simulink model "thermalBuilding3221"  (Simulink 8.3)
settings: Solver=ode5  StartTime=0.0  StopTime=24  FixedStep=stepSize  RelTol=1e-3
model workspace: external: MAT-File D:\PROGRAMMING-IDEs\MATLAB\1WORKSPACE\1_Projects\Smart-Building\WIN/Data/wsVars/thermalBuilding3221WS.mat (data not in the file)
undefined symbols (not defined in the file): Ca, Ceq, cost, DiscIntNeverNeededParam, Mafc, Mafh, Req, Rwall, stepSize, TAout, TCooler, THeater, TInit, TSet1, TSet2, TSet3
libraries: dspsigops x1
(part 1 of 2)
settings Model: Creator=salanda  LastModifiedBy=salanda
settings DataIOCC: SignalLoggingSaveFormat=Dataset
settings DebuggingCC: UnderspecifiedInitializationDetection=Simplified  ParameterPrecisionLossMsg=none  StateNameClashWarn=none
settings GRTTargetCC: CombineOutputUpdateFcns=on  GRTInterface=off

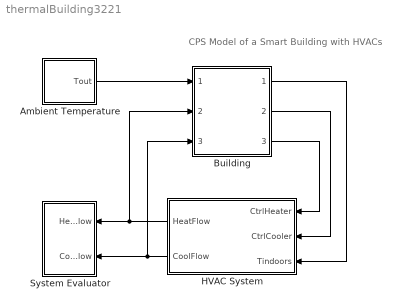
== system thermalBuilding3221 ==
  note: CPS Model of a Smart Building with HVACs
  Ambient Temperature : Subsystem
  Building : Subsystem
      mask Display: image(imread('building.png'))
  HVAC System : Subsystem
  System Evaluator : Subsystem
  wires:
  Ambient Temperature/1(Tout) -> Building/1(Outdoor Temp)
  HVAC System/1(HeatFlow) -> System Evaluator/1(HeatFlow), Building/2(HeatFlow)
  HVAC System/2(CoolFlow) -> System Evaluator/2(CoolFlow), Building/3(CoolFlow)
  Building/3(Heater  On/Off) -> HVAC System/1(CtrlHeater)
  Building/2(Cooler  On/Off) -> HVAC System/2(CtrlCooler)
  Building/1(Tindoors) -> HVAC System/3(Tindoors)

== system thermalBuilding3221/Ambient Temperature ==
  Avg Outdoor Temp : Constant  Value=TAout
  Daily Temp Variation : Sin  Amplitude=15  Frequency=2*pi/24  SampleTime=0
  Sum1 : Sum  Inputs=|++  SaturateOnIntegerOverflow=on  InputSameDT=on  OutDataTypeStr=Inherit: Same as first input
  Tout : Outport
  wires:
  Daily Temp Variation/1 -> Sum1/2
  Avg Outdoor Temp/1 -> Sum1/1
  Sum1/1 -> Tout/1

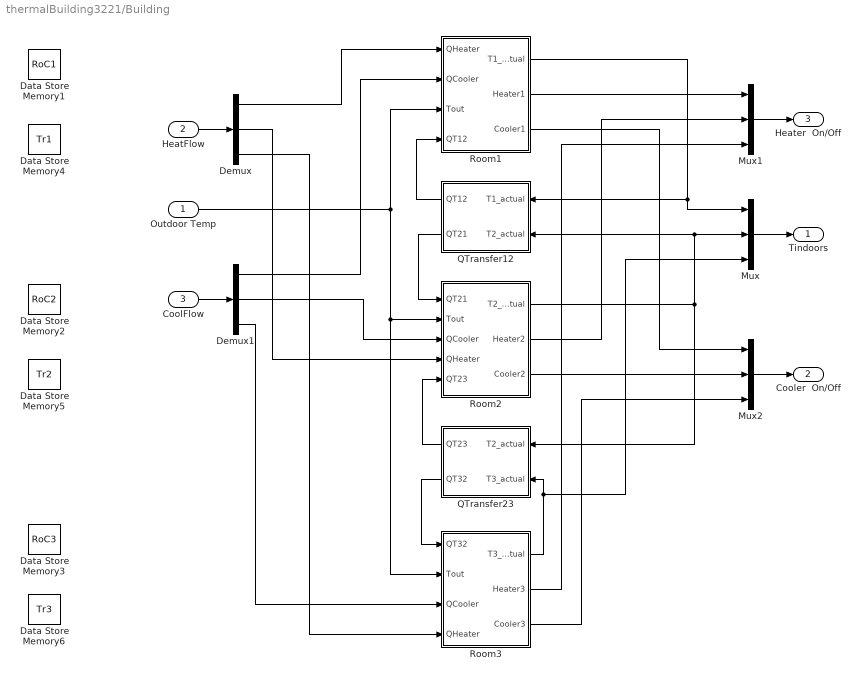
== system thermalBuilding3221/Building ==
  Outdoor Temp : Inport
  HeatFlow : Inport  Port=2
  CoolFlow : Inport  Port=3
  Data Store Memory1 : DataStoreMemory  DataStoreName=RoC1  ReadBeforeWriteMsg=warning  WriteAfterWriteMsg=warning  WriteAfterReadMsg=warning
  Data Store Memory2 : DataStoreMemory  DataStoreName=RoC2  ReadBeforeWriteMsg=warning  WriteAfterWriteMsg=warning  WriteAfterReadMsg=warning
  Data Store Memory3 : DataStoreMemory  DataStoreName=RoC3  ReadBeforeWriteMsg=warning  WriteAfterWriteMsg=warning  WriteAfterReadMsg=warning
  Data Store Memory4 : DataStoreMemory  DataStoreName=Tr1  ReadBeforeWriteMsg=warning  WriteAfterWriteMsg=warning  WriteAfterReadMsg=warning
  Data Store Memory5 : DataStoreMemory  DataStoreName=Tr2  ReadBeforeWriteMsg=warning  WriteAfterWriteMsg=warning  WriteAfterReadMsg=warning
  Data Store Memory6 : DataStoreMemory  DataStoreName=Tr3  ReadBeforeWriteMsg=warning  WriteAfterWriteMsg=warning  WriteAfterReadMsg=warning
  Demux : Demux  Outputs=3
  Demux1 : Demux  Outputs=3
  Mux : Mux  Inputs=3
  Mux1 : Mux  Inputs=3
  Mux2 : Mux  Inputs=3
  QTransfer12 : Subsystem
  QTransfer23 : Subsystem
  Room1 : Subsystem
  Room2 : Subsystem
  Room3 : Subsystem
  Tindoors : Outport
  Cooler  On/Off : Outport  Port=2
  Heater  On/Off : Outport  Port=3
  wires:
  Room1/1(T1_actual) -> QTransfer12/1(T1_actual), Mux/1
  Outdoor Temp/1 -> Room3/2(Tout), Room2/2(Tout), Room1/3(Tout)
  Demux1/1 -> Room1/2(QCooler)
  Demux/1 -> Room1/1(QHeater)
  Room1/2(Heater1) -> Mux1/1
  Room1/3(Cooler1) -> Mux2/1
  Room2/1(T2_actual) -> QTransfer12/2(T2_actual), Mux/2, QTransfer23/1(T2_actual)
  Demux1/2 -> Room2/3(QCooler)
  Demux/2 -> Room2/4(QHeater)
  Room2/2(Heater2) -> Mux1/2
  Room2/3(Cooler2) -> Mux2/2
  CoolFlow/1 -> Demux1/1
  HeatFlow/1 -> Demux/1
  Mux/1 -> Tindoors/1
  Mux1/1 -> Heater  On/Off/1
  Mux2/1 -> Cooler  On/Off/1
  QTransfer12/1(QT12) -> Room1/4(QT12)
  QTransfer12/2(QT21) -> Room2/1(QT21)
  Demux/3 -> Room3/4(QHeater)
  Demux1/3 -> Room3/3(QCooler)
  Room3/3(Cooler3) -> Mux2/3
  Room3/2(Heater3) -> Mux1/3
  QTransfer23/1(QT23) -> Room2/5(QT23)
  QTransfer23/2(QT32) -> Room3/1(QT32)
  Room3/1(T3_actual) -> Mux/3, QTransfer23/2(T3_actual)

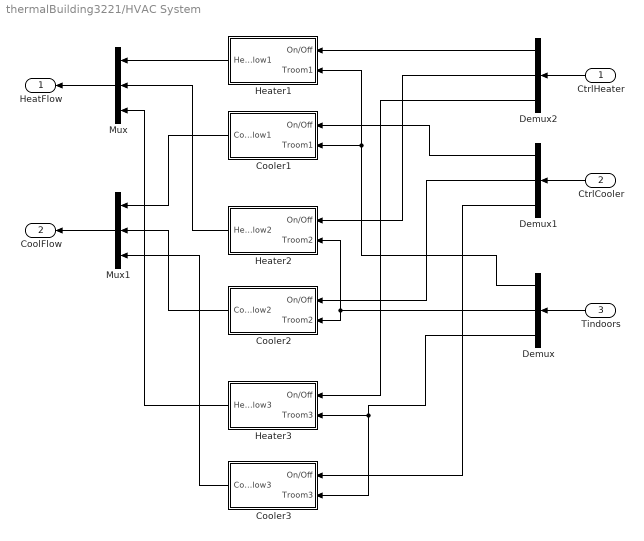
== system thermalBuilding3221/HVAC System ==
  CtrlHeater : Inport
  CtrlCooler : Inport  Port=2
  Tindoors : Inport  Port=3
  Cooler1 : Subsystem
  Cooler2 : Subsystem
  Cooler3 : Subsystem
  Demux : Demux  Outputs=3
  Demux1 : Demux  Outputs=3
  Demux2 : Demux  Outputs=3
  Heater1 : Subsystem
  Heater2 : Subsystem
  Heater3 : Subsystem
  Mux : Mux  Inputs=3
  Mux1 : Mux  Inputs=3
  HeatFlow : Outport
  CoolFlow : Outport  Port=2
  wires:
  Cooler1/1(CoolFlow1) -> Mux1/1
  Demux/1 -> Heater1/2(Troom1), Cooler1/2(Troom1)
  Demux2/1 -> Heater1/1(On/Off)
  Heater1/1(HeatFlow1) -> Mux/1
  Tindoors/1 -> Demux/1
  Demux/2 -> Cooler2/2(Troom2), Heater2/2(Troom2)
  CtrlHeater/1 -> Demux2/1
  CtrlCooler/1 -> Demux1/1
  Demux1/1 -> Cooler1/1(On/Off)
  Demux2/2 -> Heater2/1(On/Off)
  Demux1/2 -> Cooler2/1(On/Off)
  Cooler2/1(CoolFlow2) -> Mux1/2
  Heater2/1(HeatFlow2) -> Mux/2
  Mux1/1 -> CoolFlow/1
  Mux/1 -> HeatFlow/1
  Heater3/1(HeatFlow3) -> Mux/3
  Cooler3/1(CoolFlow3) -> Mux1/3
  Demux/3 -> Cooler3/2(Troom3), Heater3/2(Troom3)
  Demux2/3 -> Heater3/1(On/Off)
  Demux1/3 -> Cooler3/1(On/Off)

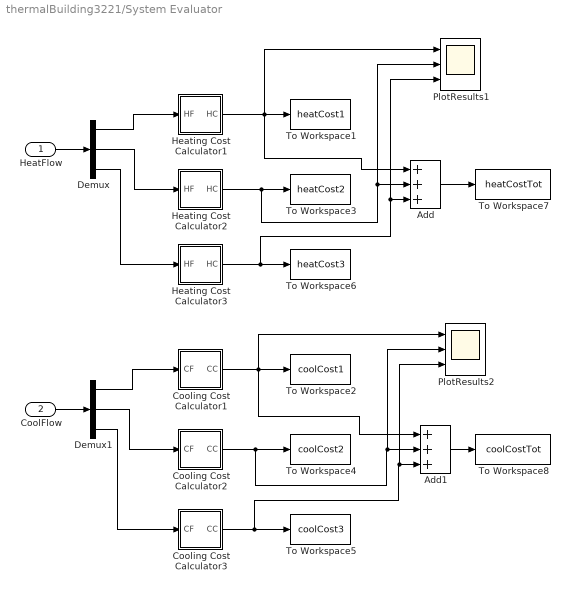
== system thermalBuilding3221/System Evaluator ==
  HeatFlow : Inport
  CoolFlow : Inport  Port=2
  Add : Sum  Inputs=+++
  Add1 : Sum  Inputs=+++
  Cooling Cost Calculator1 : Subsystem
  Cooling Cost Calculator2 : Subsystem
  Cooling Cost Calculator3 : Subsystem
  Demux : Demux  Outputs=3
  Demux1 : Demux  Outputs=3
  Heating Cost Calculator1 : Subsystem
  Heating Cost Calculator2 : Subsystem
  Heating Cost Calculator3 : Subsystem
  PlotResults1 : Scope  NumInputPorts=3
      settings: TimeRange=50  YMin=0~-5~-5  YMax=40~5~5  SaveName=a16
  PlotResults2 : Scope  NumInputPorts=3
      settings: TimeRange=50  YMin=0~-5~-5  YMax=40~5~5  SaveName=a17
  To Workspace1 : ToWorkspace  VariableName=heatCost1  SampleTime=-1
  To Workspace2 : ToWorkspace  VariableName=coolCost1  SampleTime=-1
  To Workspace3 : ToWorkspace  VariableName=heatCost2  SampleTime=-1
  To Workspace4 : ToWorkspace  VariableName=coolCost2  SampleTime=-1
  To Workspace5 : ToWorkspace  VariableName=coolCost3  SampleTime=-1
  To Workspace6 : ToWorkspace  VariableName=heatCost3  SampleTime=-1
  To Workspace7 : ToWorkspace  VariableName=heatCostTot  SampleTime=-1
  To Workspace8 : ToWorkspace  VariableName=coolCostTot  SampleTime=-1
  wires:
  Demux/1 -> Heating Cost Calculator1/1(HF)
  Demux1/1 -> Cooling Cost Calculator1/1(CF)
  Heating Cost Calculator1/1(HC) -> PlotResults1/1, Add/1, To Workspace1/1
  Cooling Cost Calculator1/1(CC) -> PlotResults2/1, Add1/1, To Workspace2/1
  HeatFlow/1 -> Demux/1
  Demux/2 -> Heating Cost Calculator2/1(HF)
  CoolFlow/1 -> Demux1/1
  Demux1/2 -> Cooling Cost Calculator2/1(CF)
  Heating Cost Calculator2/1(HC) -> Add/2, PlotResults1/2, To Workspace3/1
  Cooling Cost Calculator2/1(CC) -> PlotResults2/2, Add1/2, To Workspace4/1
  Cooling Cost Calculator3/1(CC) -> PlotResults2/3, Add1/3, To Workspace5/1
  Heating Cost Calculator3/1(HC) -> PlotResults1/3, Add/3, To Workspace6/1
  Demux/3 -> Heating Cost Calculator3/1(HF)
  Demux1/3 -> Cooling Cost Calculator3/1(CF)
  Add/1 -> To Workspace7/1
  Add1/1 -> To Workspace8/1

== system thermalBuilding3221/Building/QTransfer12 ==
  note: T1 - T2
  note: T2 - T1
  T1_actual : Inport
  T2_actual : Inport  Port=2
  Multiport Switch : MultiPortSwitch  DataPortOrder=Zero-based contiguous  Inputs=2
  RO : RelationalOperator  Operator=<=  OutDataTypeStr=boolean
  Subtract1 : Sum  Inputs=+-
  Subtract2 : Sum  Inputs=+-
  Ther Res1 : Gain  Gain=(1/Rwall)*(1/4)  SaturateOnIntegerOverflow=on  OutDataTypeStr=Inherit: Same as input  ParamDataTypeStr=Inherit: Same as input
  Ther Res2 : Gain  Gain=(1/Rwall)*(1/4)  SaturateOnIntegerOverflow=on  OutDataTypeStr=Inherit: Same as input  ParamDataTypeStr=Inherit: Same as input
  Unary Minus : UnaryMinus
  QT12 : Outport
  QT21 : Outport  Port=2
  wires:
  T1_actual/1 -> RO/1, Subtract1/1, Subtract2/2
  RO/1 -> Multiport Switch/1
  Subtract1/1 -> Ther Res1/1
  Ther Res1/1 -> Multiport Switch/2
  Subtract2/1 -> Ther Res2/1
  T2_actual/1 -> Subtract1/2, Subtract2/1, RO/2
  Ther Res2/1 -> Multiport Switch/3
  Multiport Switch/1 -> Unary Minus/1, QT12/1
  Unary Minus/1 -> QT21/1

== system thermalBuilding3221/Building/QTransfer23 ==
  note: T2 - T3
  note: T3 - T2
  T2_actual : Inport
  T3_actual : Inport  Port=2
  Multiport Switch : MultiPortSwitch  DataPortOrder=Zero-based contiguous  Inputs=2
  RO : RelationalOperator  Operator=<=  OutDataTypeStr=boolean
  Subtract1 : Sum  Inputs=+-
  Subtract2 : Sum  Inputs=+-
  Ther Res1 : Gain  Gain=(1/Rwall)*(1/4)  SaturateOnIntegerOverflow=on  OutDataTypeStr=Inherit: Same as input  ParamDataTypeStr=Inherit: Same as input
  Ther Res2 : Gain  Gain=(1/Rwall)*(1/4)  SaturateOnIntegerOverflow=on  OutDataTypeStr=Inherit: Same as input  ParamDataTypeStr=Inherit: Same as input
  Unary Minus : UnaryMinus
  QT23 : Outport
  QT32 : Outport  Port=2
  wires:
  T2_actual/1 -> RO/1, Subtract1/1, Subtract2/2
  RO/1 -> Multiport Switch/1
  Subtract1/1 -> Ther Res1/1
  Ther Res1/1 -> Multiport Switch/2
  Subtract2/1 -> Ther Res2/1
  T3_actual/1 -> Subtract1/2, Subtract2/1, RO/2
  Ther Res2/1 -> Multiport Switch/3
  Multiport Switch/1 -> Unary Minus/1, QT23/1
  Unary Minus/1 -> QT32/1

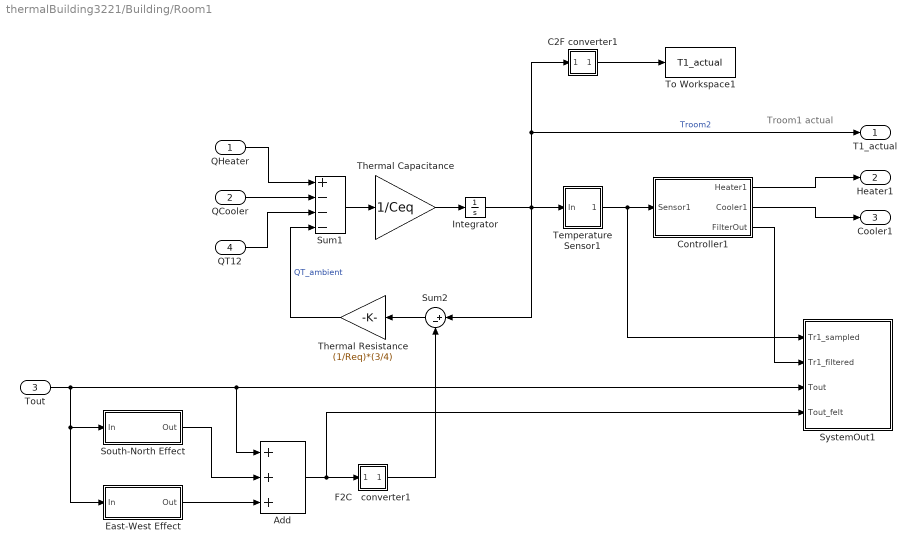
== system thermalBuilding3221/Building/Room1 ==
  note: Troom1 actual
  QHeater : Inport
  QCooler : Inport  Port=2
  Tout : Inport  Port=3
  QT12 : Inport  Port=4
  Add : Sum  Inputs=+++
  C2F converter1 : Subsystem  mask(F2C){}
      mask help:
      | Conversion from degrees Fahrenheit to degrees Celsius.
      |
      | F = C * (9/5) + 32;
      mask Display: image(imread('fahrenheit.jpg'))
  Controller1 : Subsystem
      mask help: the controller is used to trigger the heater when the room temp drops below a reference temperature and to trigger the cooler when the room temp raises above the reference temperature.
      mask Display: image(imread('RaspberryPi2_mod.jpg'))
  East-West Effect : Subsystem
  F2C   converter1 : Subsystem  mask(F2C){}
      mask help:
      | Conversion from degrees Fahrenheit to degrees Celsius.
      |
      | C = (F-32) * (5/9);
      mask Display: image(imread('celsius.jpg'))
  Integrator : Integrator  InitialCondition=(TInit-32)*5/9
  South-North Effect : Subsystem
  Sum1 : Sum  Inputs=+---  SaturateOnIntegerOverflow=on  InputSameDT=on  OutDataTypeStr=Inherit: Same as first input
  Sum2 : Sum  Inputs=|+-  SaturateOnIntegerOverflow=on  InputSameDT=on  OutDataTypeStr=Inherit: Same as first input
  SystemOut1 : Subsystem
  Temperature Sensor1 : Subsystem  mask(Building Thermostat){}
      mask help: The temperature sensor is used to provide data samples for indoor temperature.
      mask Display: image(fullfile(matlabroot,'toolbox','simulink','simdemos','simgeneral','images','HouseHeatThermostatPix.svg'))
  Thermal Capacitance : Gain  Gain=1/Ceq  SaturateOnIntegerOverflow=on  OutDataTypeStr=Inherit: Same as input  ParamDataTypeStr=Inherit: Same as input
  Thermal Resistance : Gain  Gain=(1/Req)*(3/4)  SaturateOnIntegerOverflow=on  OutDataTypeStr=Inherit: Same as input  ParamDataTypeStr=Inherit: Same as input
  To Workspace1 : ToWorkspace  VariableName=T1_actual  SampleTime=-1
  T1_actual : Outport
  Heater1 : Outport  Port=2
  Cooler1 : Outport  Port=3
  wires:
  Thermal Resistance/1 -> Sum1/4  "QT_ambient"
  Thermal Capacitance/1 -> Integrator/1
  QHeater/1 -> Sum1/1
  Sum1/1 -> Thermal Capacitance/1
  Sum2/1 -> Thermal Resistance/1
  F2C   converter1/1(C) -> Sum2/2
  QCooler/1 -> Sum1/2
  Add/1 -> SystemOut1/4(Tout_felt), F2C   converter1/1(F)
  QT12/1 -> Sum1/3
  South-North Effect/1(Out) -> Add/2
  East-West Effect/1(Out) -> Add/3
  Tout/1 -> SystemOut1/3(Tout), Add/1, East-West Effect/1(In), South-North Effect/1(In)
  Controller1/1(Heater1) -> Heater1/1
  Controller1/2(Cooler1) -> Cooler1/1
  Temperature Sensor1/1(Out) -> SystemOut1/1(Tr1_sampled), Controller1/1(Sensor1)
  Controller1/3(FilterOut) -> SystemOut1/2(Tr1_filtered)
  Integrator/1 -> T1_actual/1, C2F converter1/1(F), Temperature Sensor1/1(In), Sum2/1  "Troom2"
  C2F converter1/1(C) -> To Workspace1/1

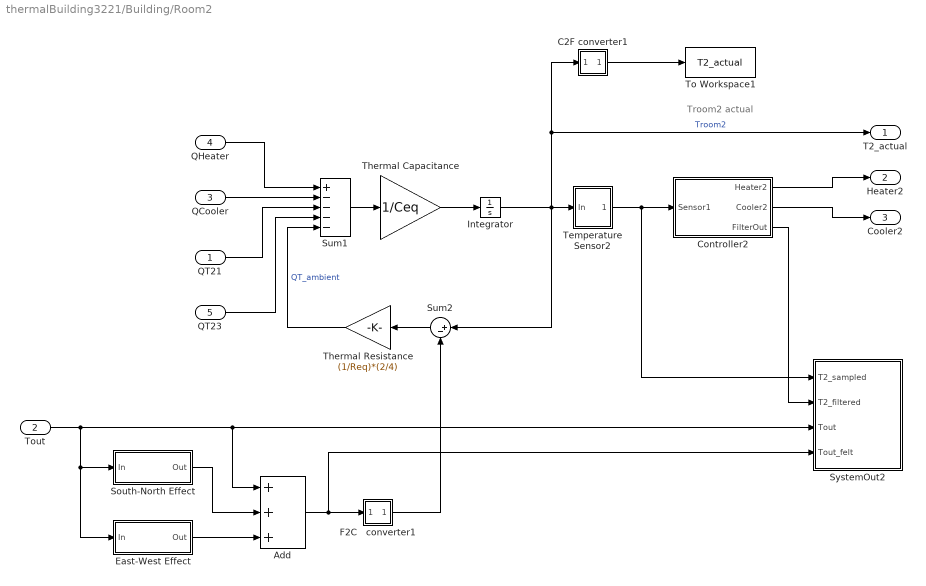
== system thermalBuilding3221/Building/Room2 ==
  note: Troom2 actual
  QT21 : Inport
  Tout : Inport  Port=2
  QCooler : Inport  Port=3
  QHeater : Inport  Port=4
  QT23 : Inport  Port=5
  Add : Sum  Inputs=+++
  C2F converter1 : Subsystem  mask(F2C){}
      mask help:
      | Conversion from degrees Fahrenheit to degrees Celsius.
      |
      | F = C * (9/5) + 32;
      mask Display: image(imread('fahrenheit.jpg'))
  Controller2 : Subsystem
      mask help: the controller is used to trigger the heater when the room temp drops below a reference temperature and to trigger the cooler when the room temp raises above the reference temperature.
      mask Display: image(imread('RaspberryPi2_mod.jpg'))
  East-West Effect : Subsystem
  F2C   converter1 : Subsystem  mask(F2C){}
      mask help:
      | Conversion from degrees Fahrenheit to degrees Celsius.
      |
      | C = (F-32) * (5/9);
      mask Display: image(imread('celsius.jpg'))
  Integrator : Integrator  InitialCondition=(TInit-32)*5/9
  South-North Effect : Subsystem
  Sum1 : Sum  Inputs=+----  SaturateOnIntegerOverflow=on  InputSameDT=on  OutDataTypeStr=Inherit: Same as first input
  Sum2 : Sum  Inputs=|+-  SaturateOnIntegerOverflow=on  InputSameDT=on  OutDataTypeStr=Inherit: Same as first input
  SystemOut2 : Subsystem
  Temperature Sensor2 : Subsystem  mask(Building Thermostat){}
      mask help: The temperature sensor is used to provide data samples for indoor temperature.
      mask Display: image(fullfile(matlabroot,'toolbox','simulink','simdemos','simgeneral','images','HouseHeatThermostatPix.svg'))
  Thermal Capacitance : Gain  Gain=1/Ceq  SaturateOnIntegerOverflow=on  OutDataTypeStr=Inherit: Same as input  ParamDataTypeStr=Inherit: Same as input
  Thermal Resistance : Gain  Gain=(1/Req)*(2/4)  SaturateOnIntegerOverflow=on  OutDataTypeStr=Inherit: Same as input  ParamDataTypeStr=Inherit: Same as input
  To Workspace1 : ToWorkspace  VariableName=T2_actual  SampleTime=-1
  T2_actual : Outport
  Heater2 : Outport  Port=2
  Cooler2 : Outport  Port=3
  wires:
  Thermal Resistance/1 -> Sum1/5  "QT_ambient"
  Thermal Capacitance/1 -> Integrator/1
  QHeater/1 -> Sum1/1
  Sum1/1 -> Thermal Capacitance/1
  Sum2/1 -> Thermal Resistance/1
  F2C   converter1/1(C) -> Sum2/2
  QCooler/1 -> Sum1/2
  Add/1 -> SystemOut2/4(Tout_felt), F2C   converter1/1(F)
  Temperature Sensor2/1(Out) -> SystemOut2/1(T2_sampled), Controller2/1(Sensor1)
  QT21/1 -> Sum1/3
  QT23/1 -> Sum1/4
  South-North Effect/1(Out) -> Add/2
  East-West Effect/1(Out) -> Add/3
  Tout/1 -> SystemOut2/3(Tout), Add/1, East-West Effect/1(In), South-North Effect/1(In)
  Controller2/1(Heater2) -> Heater2/1
  Controller2/2(Cooler2) -> Cooler2/1
  Controller2/3(FilterOut) -> SystemOut2/2(T2_filtered)
  Integrator/1 -> C2F converter1/1(F), T2_actual/1, Temperature Sensor2/1(In), Sum2/1  "Troom2"
  C2F converter1/1(C) -> To Workspace1/1

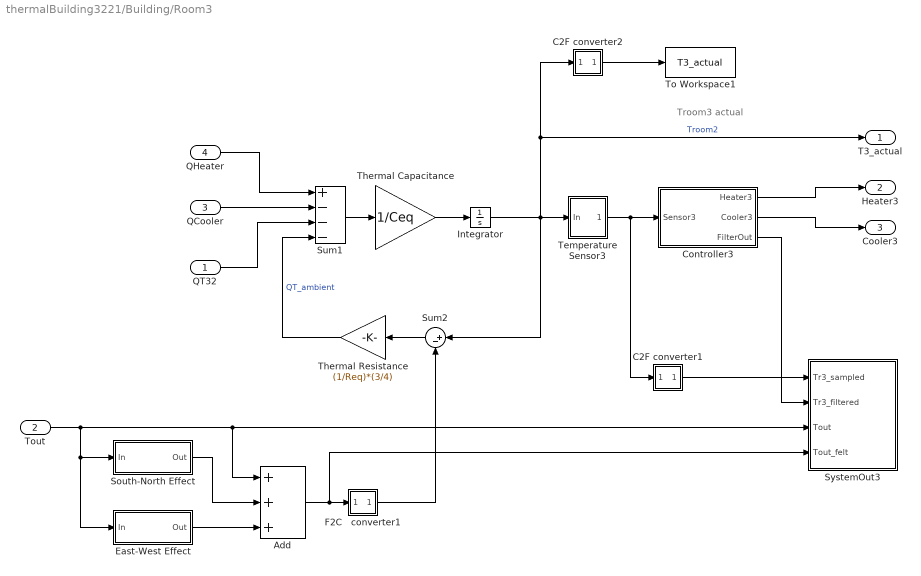
== system thermalBuilding3221/Building/Room3 ==
  note: Troom3 actual
  QT32 : Inport
  Tout : Inport  Port=2
  QCooler : Inport  Port=3
  QHeater : Inport  Port=4
  Add : Sum  Inputs=+++
  C2F converter1 : Subsystem  mask(F2C){}
      mask help:
      | Conversion from degrees Fahrenheit to degrees Celsius.
      |
      | F = C * (9/5) + 32;
      mask Display: image(imread('fahrenheit.jpg'))
  C2F converter2 : Subsystem  mask(F2C){}
      mask help:
      | Conversion from degrees Fahrenheit to degrees Celsius.
      |
      | F = C * (9/5) + 32;
      mask Display: image(imread('fahrenheit.jpg'))
  Controller3 : Subsystem
      mask help: the controller is used to trigger the heater when the room temp drops below a reference temperature and to trigger the cooler when the room temp raises above the reference temperature.
      mask Display: image(imread('RaspberryPi2_mod.jpg'))
  East-West Effect : Subsystem
  F2C   converter1 : Subsystem  mask(F2C){}
      mask help:
      | Conversion from degrees Fahrenheit to degrees Celsius.
      |
      | C = (F-32) * (5/9);
      mask Display: image(imread('celsius.jpg'))
  Integrator : Integrator  InitialCondition=(TInit-32)*5/9
  South-North Effect : Subsystem
  Sum1 : Sum  Inputs=+---  SaturateOnIntegerOverflow=on  InputSameDT=on  OutDataTypeStr=Inherit: Same as first input
  Sum2 : Sum  Inputs=|+-  SaturateOnIntegerOverflow=on  InputSameDT=on  OutDataTypeStr=Inherit: Same as first input
  SystemOut3 : Subsystem
  "Temperature Sensor3 " : Subsystem  mask(Building Thermostat){}
      mask help: The temperature sensor is used to provide data samples for indoor temperature.
      mask Display: image(fullfile(matlabroot,'toolbox','simulink','simdemos','simgeneral','images','HouseHeatThermostatPix.svg'))
  Thermal Capacitance : Gain  Gain=1/Ceq  SaturateOnIntegerOverflow=on  OutDataTypeStr=Inherit: Same as input  ParamDataTypeStr=Inherit: Same as input
  Thermal Resistance : Gain  Gain=(1/Req)*(3/4)  SaturateOnIntegerOverflow=on  OutDataTypeStr=Inherit: Same as input  ParamDataTypeStr=Inherit: Same as input
  To Workspace1 : ToWorkspace  VariableName=T3_actual  SampleTime=-1
  T3_actual : Outport
  Heater3 : Outport  Port=2
  Cooler3 : Outport  Port=3
  wires:
  Thermal Resistance/1 -> Sum1/4  "QT_ambient"
  Thermal Capacitance/1 -> Integrator/1
  QHeater/1 -> Sum1/1
  Sum1/1 -> Thermal Capacitance/1
  Sum2/1 -> Thermal Resistance/1
  F2C   converter1/1(C) -> Sum2/2
  QCooler/1 -> Sum1/2
  Add/1 -> SystemOut3/4(Tout_felt), F2C   converter1/1(F)
  C2F converter1/1(C) -> SystemOut3/1(Tr3_sampled)
  QT32/1 -> Sum1/3
  South-North Effect/1(Out) -> Add/2
  East-West Effect/1(Out) -> Add/3
  Tout/1 -> Add/1, SystemOut3/3(Tout), East-West Effect/1(In), South-North Effect/1(In)
  "Temperature Sensor3 "/1(Out) -> Controller3/1(Sensor3), C2F converter1/1(F)
  Controller3/1(Heater3) -> Heater3/1
  Controller3/2(Cooler3) -> Cooler3/1
  Controller3/3(FilterOut) -> SystemOut3/2(Tr3_filtered)
  Integrator/1 -> C2F converter2/1(F), T3_actual/1, "Temperature Sensor3 "/1(In), Sum2/1  "Troom2"
  C2F converter2/1(C) -> To Workspace1/1

== system thermalBuilding3221/HVAC System/Cooler1 ==
  note: Control Command (On/Off)
  note: Cooling Facility of HVAC System
  On/Off : Inport
  Troom1 : Inport  Port=2
  Cooler Air Temperature : Constant  Value=TCooler
  Cooler Switch : Product  RndMeth=Zero
  F2C   converter1 : Subsystem  mask(F2C){}
      mask help:
      | Conversion from degrees Fahrenheit to degrees Celsius.
      |
      | C = (F-32) * (5/9);
      mask Display: image(imread('celsius.jpg'))
  HeatGain : Gain  Gain=Mafc*Ca
  Plot : Scope
      settings: TickLabels=on  ShowLegends=on  TimeRange=50  YMin=0  YMax=40  SaveName=a3
  Sum2 : Sum  Inputs=|+-
  CoolFlow1 : Outport
  wires:
  Cooler Switch/1 -> CoolFlow1/1
  HeatGain/1 -> Cooler Switch/2
  On/Off/1 -> Plot/1, Cooler Switch/1
  Sum2/1 -> HeatGain/1
  Troom1/1 -> Sum2/1
  Cooler Air Temperature/1 -> F2C   converter1/1(F)
  F2C   converter1/1(C) -> Sum2/2

== system thermalBuilding3221/HVAC System/Cooler2 ==
  note: Control Command (On/Off)
  note: Cooling Facility of HVAC System
  On/Off : Inport
  Troom2 : Inport  Port=2
  Cooler Air Temperature : Constant  Value=TCooler
  Cooler Switch : Product  RndMeth=Zero
  F2C   converter1 : Subsystem  mask(F2C){}
      mask help:
      | Conversion from degrees Fahrenheit to degrees Celsius.
      |
      | C = (F-32) * (5/9);
      mask Display: image(imread('celsius.jpg'))
  HeatGain : Gain  Gain=Mafc*Ca
  Plot : Scope
      settings: TickLabels=on  ShowLegends=on  TimeRange=50  YMin=0  YMax=40  SaveName=a3
  Sum2 : Sum  Inputs=|+-
  CoolFlow2 : Outport
  wires:
  Cooler Air Temperature/1 -> F2C   converter1/1(F)
  Troom2/1 -> Sum2/1
  Sum2/1 -> HeatGain/1
  On/Off/1 -> Cooler Switch/1, Plot/1
  HeatGain/1 -> Cooler Switch/2
  Cooler Switch/1 -> CoolFlow2/1
  F2C   converter1/1(C) -> Sum2/2

== system thermalBuilding3221/HVAC System/Cooler3 ==
  note: Control Command (On/Off)
  note: Cooling Facility of HVAC System
  On/Off : Inport
  Troom3 : Inport  Port=2
  Cooler Air Temperature : Constant  Value=TCooler
  Cooler Switch : Product  RndMeth=Zero
  F2C   converter1 : Subsystem  mask(F2C){}
      mask help:
      | Conversion from degrees Fahrenheit to degrees Celsius.
      |
      | C = (F-32) * (5/9);
      mask Display: image(imread('celsius.jpg'))
  HeatGain : Gain  Gain=Mafc*Ca
  Plot : Scope
      settings: TickLabels=on  ShowLegends=on  TimeRange=50  YMin=0  YMax=40  SaveName=a3
  Sum2 : Sum  Inputs=|+-
  CoolFlow3 : Outport
  wires:
  Cooler Air Temperature/1 -> F2C   converter1/1(F)
  Troom3/1 -> Sum2/1
  Sum2/1 -> HeatGain/1
  On/Off/1 -> Cooler Switch/1, Plot/1
  HeatGain/1 -> Cooler Switch/2
  Cooler Switch/1 -> CoolFlow3/1
  F2C   converter1/1(C) -> Sum2/2

== system thermalBuilding3221/HVAC System/Heater1 ==
  note: Heating Facility of HVAC System
  On/Off : Inport
  Troom1 : Inport  Port=2
  F2C   converter1 : Subsystem  mask(F2C){}
      mask help:
      | Conversion from degrees Fahrenheit to degrees Celsius.
      |
      | C = (F-32) * (5/9);
      mask Display: image(imread('celsius.jpg'))
  HeatGain : Gain  Gain=Mafh*Ca
  Heater Air Temperature : Constant  Value=THeater
  Heater Switch : Product  RndMeth=Zero
  Plot : Scope
      settings: TickLabels=on  ShowLegends=on  TimeRange=50  YMin=0  YMax=40  SaveName=a2
  Sum2 : Sum  Inputs=|-+
  HeatFlow1 : Outport
  wires:
  Heater Air Temperature/1 -> F2C   converter1/1(F)
  Troom1/1 -> Sum2/1
  Sum2/1 -> HeatGain/1
  On/Off/1 -> Plot/1, Heater Switch/1  "Control Command (On/Off)"
  HeatGain/1 -> Heater Switch/2
  Heater Switch/1 -> HeatFlow1/1
  F2C   converter1/1(C) -> Sum2/2

== system thermalBuilding3221/HVAC System/Heater2 ==
  note: Heating Facility of HVAC System
  On/Off : Inport
  Troom2 : Inport  Port=2
  F2C   converter1 : Subsystem  mask(F2C){}
      mask help:
      | Conversion from degrees Fahrenheit to degrees Celsius.
      |
      | C = (F-32) * (5/9);
      mask Display: image(imread('celsius.jpg'))
  HeatGain : Gain  Gain=Mafh*Ca
  Heater Air Temperature : Constant  Value=THeater
  Heater Switch : Product  RndMeth=Zero
  Plot : Scope
      settings: TickLabels=on  ShowLegends=on  TimeRange=50  YMin=0  YMax=40  SaveName=a2
  Sum2 : Sum  Inputs=|-+
  HeatFlow2 : Outport
  wires:
  Heater Switch/1 -> HeatFlow2/1
  HeatGain/1 -> Heater Switch/2
  On/Off/1 -> Plot/1, Heater Switch/1  "Control Command (On/Off)"
  Sum2/1 -> HeatGain/1
  Troom2/1 -> Sum2/1
  Heater Air Temperature/1 -> F2C   converter1/1(F)
  F2C   converter1/1(C) -> Sum2/2

== system thermalBuilding3221/HVAC System/Heater3 ==
  note: Heating Facility of HVAC System
  On/Off : Inport
  Troom3 : Inport  Port=2
  F2C   converter1 : Subsystem  mask(F2C){}
      mask help:
      | Conversion from degrees Fahrenheit to degrees Celsius.
      |
      | C = (F-32) * (5/9);
      mask Display: image(imread('celsius.jpg'))
  HeatGain : Gain  Gain=Mafh*Ca
  Heater Air Temperature : Constant  Value=THeater
  Heater Switch : Product  RndMeth=Zero
  Plot : Scope
      settings: TickLabels=on  ShowLegends=on  TimeRange=50  YMin=0  YMax=40  SaveName=a2
  Sum2 : Sum  Inputs=|-+
  HeatFlow3 : Outport
  wires:
  Heater Switch/1 -> HeatFlow3/1
  HeatGain/1 -> Heater Switch/2
  On/Off/1 -> Heater Switch/1, Plot/1  "Control Command (On/Off)"
  Sum2/1 -> HeatGain/1
  Troom3/1 -> Sum2/1
  Heater Air Temperature/1 -> F2C   converter1/1(F)
  F2C   converter1/1(C) -> Sum2/2

== system thermalBuilding3221/System Evaluator/Cooling Cost Calculator1 ==
  CF : Inport
  Cost  Coefficient : Gain  Gain=cost  SaturateOnIntegerOverflow=on  OutDataTypeStr=Inherit: Same as input  ParamDataTypeStr=Inherit: Same as input
  Divide : Product  Inputs=*/
  Divide1 : Product  Inputs=*/
  Integrator : Integrator
  J2kWh : Constant  Value=3.6e6
  J2kWh1 : Constant  Value=3.6e6
  PlotResults1 : Scope  NumInputPorts=2
      settings: TimeRange=50  YMin=0~-5  YMax=40~5  SaveName=a10
  PlotResults2 : Scope  NumInputPorts=2
      settings: TimeRange=50  YMin=0~-5  YMax=40~5  SaveName=a11
  To Workspace : ToWorkspace  VariableName=Qcool1tot  SampleTime=-1
  To Workspace1 : ToWorkspace  VariableName=Qcool1  SampleTime=-1
  CC : Outport
  wires:
  Cost  Coefficient/1 -> CC/1  "CoolingCost"
  J2kWh/1 -> Divide/2
  Divide/1 -> To Workspace/1, PlotResults1/2
  Divide1/1 -> To Workspace1/1, PlotResults2/2
  J2kWh1/1 -> Divide1/2
  Integrator/1 -> Divide/1, PlotResults1/1, Cost  Coefficient/1
  CF/1 -> PlotResults2/1, Divide1/1, Integrator/1

== system thermalBuilding3221/System Evaluator/Cooling Cost Calculator2 ==
  CF : Inport
  Cost  Coefficient : Gain  Gain=cost  SaturateOnIntegerOverflow=on  OutDataTypeStr=Inherit: Same as input  ParamDataTypeStr=Inherit: Same as input
  Divide : Product  Inputs=*/
  Divide1 : Product  Inputs=*/
  Integrator : Integrator
  J2kWh : Constant  Value=3.6e6
  J2kWh1 : Constant  Value=3.6e6
  PlotResults1 : Scope  NumInputPorts=2
      settings: TimeRange=50  YMin=0~-5  YMax=40~5  SaveName=a4
  PlotResults2 : Scope  NumInputPorts=2
      settings: TimeRange=50  YMin=0~-5  YMax=40~5  SaveName=a7
  To Workspace : ToWorkspace  VariableName=Qcool2tot  SampleTime=-1
  To Workspace1 : ToWorkspace  VariableName=Qcool2  SampleTime=-1
  CC : Outport
  wires:
  Cost  Coefficient/1 -> CC/1  "CoolingCost"
  Integrator/1 -> PlotResults1/1, Divide/1, Cost  Coefficient/1
  Divide/1 -> PlotResults1/2, To Workspace/1
  J2kWh/1 -> Divide/2
  CF/1 -> PlotResults2/1, Divide1/1, Integrator/1
  Divide1/1 -> To Workspace1/1, PlotResults2/2
  J2kWh1/1 -> Divide1/2

== system thermalBuilding3221/System Evaluator/Cooling Cost Calculator3 ==
  CF : Inport
  Cost  Coefficient : Gain  Gain=cost  SaturateOnIntegerOverflow=on  OutDataTypeStr=Inherit: Same as input  ParamDataTypeStr=Inherit: Same as input
  Divide : Product  Inputs=*/
  Divide1 : Product  Inputs=*/
  Integrator : Integrator
  J2kWh : Constant  Value=3.6e6
  J2kWh1 : Constant  Value=3.6e6
  PlotResults1 : Scope  NumInputPorts=2
      settings: TimeRange=50  YMin=0~-5  YMax=40~5  SaveName=a14
  PlotResults2 : Scope  NumInputPorts=2
      settings: TimeRange=50  YMin=0~-5  YMax=40~5  SaveName=a15
  To Workspace : ToWorkspace  VariableName=Qcool3tot  SampleTime=-1
  To Workspace1 : ToWorkspace  VariableName=Qcool3  SampleTime=-1
  CC : Outport
  wires:
  Cost  Coefficient/1 -> CC/1  "CoolingCost"
  Integrator/1 -> PlotResults1/1, Divide/1, Cost  Coefficient/1
  Divide/1 -> PlotResults1/2, To Workspace/1
  J2kWh/1 -> Divide/2
  CF/1 -> PlotResults2/1, Divide1/1, Integrator/1
  Divide1/1 -> To Workspace1/1, PlotResults2/2
  J2kWh1/1 -> Divide1/2

== system thermalBuilding3221/System Evaluator/Heating Cost Calculator1 ==
  HF : Inport
  Cost  Coefficient : Gain  Gain=cost  SaturateOnIntegerOverflow=on  OutDataTypeStr=Inherit: Same as input  ParamDataTypeStr=Inherit: Same as input
  Divide : Product  Inputs=*/
  Divide1 : Product  Inputs=*/
  Integrator : Integrator
  J2kWh : Constant  Value=3.6e6
  J2kWh1 : Constant  Value=3.6e6
  PlotResults1 : Scope  NumInputPorts=2
      settings: TimeRange=50  YMin=0~-5  YMax=40~5  SaveName=a8
  PlotResults2 : Scope  NumInputPorts=2
      settings: TimeRange=50  YMin=0~-5  YMax=40~5  SaveName=a9
  To Workspace : ToWorkspace  VariableName=Qheat1tot  SampleTime=-1
  To Workspace1 : ToWorkspace  VariableName=Qheat1  SampleTime=-1
  HC : Outport
  wires:
  Cost  Coefficient/1 -> HC/1  "HeatCost"
  J2kWh/1 -> Divide/2
  Divide/1 -> To Workspace/1, PlotResults1/2
  Divide1/1 -> To Workspace1/1, PlotResults2/2
  J2kWh1/1 -> Divide1/2
  Integrator/1 -> Divide/1, PlotResults1/1, Cost  Coefficient/1
  HF/1 -> PlotResults2/1, Divide1/1, Integrator/1

== system thermalBuilding3221/System Evaluator/Heating Cost Calculator2 ==
  HF : Inport
  Cost  Coefficient : Gain  Gain=cost  SaturateOnIntegerOverflow=on  OutDataTypeStr=Inherit: Same as input  ParamDataTypeStr=Inherit: Same as input
  Divide : Product  Inputs=*/
  Divide1 : Product  Inputs=*/
  Integrator : Integrator
  J2kWh : Constant  Value=3.6e6
  J2kWh1 : Constant  Value=3.6e6
  PlotResults1 : Scope  NumInputPorts=2
      settings: TimeRange=50  YMin=0~-5  YMax=40~5  SaveName=a6
  PlotResults2 : Scope  NumInputPorts=2
      settings: TimeRange=50  YMin=0~-5  YMax=40~5  SaveName=a5
  To Workspace : ToWorkspace  VariableName=Qheat2tot  SampleTime=-1
  To Workspace1 : ToWorkspace  VariableName=Qheat2  SampleTime=-1
  HC : Outport
  wires:
  Cost  Coefficient/1 -> HC/1  "HeatCost"
  Integrator/1 -> PlotResults1/1, Divide/1, Cost  Coefficient/1
  J2kWh/1 -> Divide/2
  Divide/1 -> To Workspace/1, PlotResults1/2
  HF/1 -> PlotResults2/1, Divide1/1, Integrator/1
  Divide1/1 -> To Workspace1/1, PlotResults2/2
  J2kWh1/1 -> Divide1/2

== system thermalBuilding3221/System Evaluator/Heating Cost Calculator3 ==
  HF : Inport
  Cost  Coefficient : Gain  Gain=cost  SaturateOnIntegerOverflow=on  OutDataTypeStr=Inherit: Same as input  ParamDataTypeStr=Inherit: Same as input
  Divide : Product  Inputs=*/
  Divide1 : Product  Inputs=*/
  Integrator : Integrator
  J2kWh : Constant  Value=3.6e6
  J2kWh1 : Constant  Value=3.6e6
  PlotResults1 : Scope  NumInputPorts=2
      settings: TimeRange=50  YMin=0~-5  YMax=40~5  SaveName=a12
  PlotResults2 : Scope  NumInputPorts=2
      settings: TimeRange=50  YMin=0~-5  YMax=40~5  SaveName=a13
  To Workspace : ToWorkspace  VariableName=Qheat3tot  SampleTime=-1
  To Workspace1 : ToWorkspace  VariableName=Qheat3  SampleTime=-1
  HC : Outport
  wires:
  Cost  Coefficient/1 -> HC/1  "HeatCost"
  Integrator/1 -> PlotResults1/1, Divide/1, Cost  Coefficient/1
  J2kWh/1 -> Divide/2
  Divide/1 -> To Workspace/1, PlotResults1/2
  HF/1 -> PlotResults2/1, Divide1/1, Integrator/1
  Divide1/1 -> To Workspace1/1, PlotResults2/2
  J2kWh1/1 -> Divide1/2

== system thermalBuilding3221/Building/Room1/C2F converter1 ==
  F : Inport
  Constant1 : Constant  Value=32  OutDataTypeStr=Inherit: Inherit via back propagation
  Gain : Gain  Gain=9/5  SaturateOnIntegerOverflow=on  OutDataTypeStr=Inherit: Same as input  ParamDataTypeStr=Inherit: Same as input
  Sum1 : Sum  SaturateOnIntegerOverflow=on  InputSameDT=on  OutDataTypeStr=Inherit: Same as first input
  C : Outport
  wires:
  F/1 -> Gain/1
  Gain/1 -> Sum1/1
  Sum1/1 -> C/1
  Constant1/1 -> Sum1/2

== system thermalBuilding3221/Building/Room1/Controller1 ==
  note: Controller Subsystem
  note: Tset - Troom
  Sensor1 : Inport
  Data Store Write1 : DataStoreWrite  DataStoreName=RoC1
  Data Store Write2 : DataStoreWrite  DataStoreName=Tr1
  Negate : UnaryMinus
  Reference Temperature : Subsystem
  Relay1 : Relay  OnSwitchValue=5*(5/9)  OffSwitchValue=0
  Relay2 : Relay  OnSwitchValue=5*(5/9)  OffSwitchValue=0
  RoC1 : Subsystem
  Sum : Sum  Inputs=-+|  SaturateOnIntegerOverflow=on  InputSameDT=on  OutDataTypeStr=Inherit: Same as first input
  Heater1 : Outport
  Cooler1 : Outport  Port=2
  FilterOut : Outport  Port=3
  wires:
  Reference Temperature/1(Tset) -> Sum/2
  Relay1/1 -> Heater1/1
  Relay2/1 -> Cooler1/1
  Negate/1 -> Relay2/1
  Sum/1 -> Relay1/1, Negate/1  "Tdiff"
  Sensor1/1 -> Sum/1, Data Store Write2/1, FilterOut/1, RoC1/1(In1)
  RoC1/1(Out1) -> Data Store Write1/1

== system thermalBuilding3221/Building/Room1/East-West Effect ==
  note: 0: West
      | 1: East
      | 2: Both / No
  note: Room Orientation East-West
  In : Inport
  Both / No Direction : Constant  Value=0
  Constant1 : Constant  Value=0.05
  East-West : Constant  Value=0
  From Workspace1 : FromWorkspace  VariableName=east  SampleTime=0
  From Workspace2 : FromWorkspace  VariableName=west  SampleTime=0
  Multiport Switch1 : MultiPortSwitch  DataPortOrder=Specify indices  Inputs=2  DataPortIndices={1,0,2}  DiagnosticForDefault=None
  Product1 : Product  Inputs=3
  Scope : Scope  NumInputPorts=2
      settings: YMin=-5~-5  YMax=5~5
  Out : Outport
  wires:
  From Workspace1/1 -> Scope/1, Multiport Switch1/2
  East-West/1 -> Multiport Switch1/1
  Product1/1 -> Out/1
  From Workspace2/1 -> Scope/2, Multiport Switch1/3
  Both / No Direction/1 -> Multiport Switch1/4
  Constant1/1 -> Product1/2
  In/1 -> Product1/3
  Multiport Switch1/1 -> Product1/1

== system thermalBuilding3221/Building/Room1/F2C   converter1 ==
  F : Inport
  Constant : Constant  Value=32  OutDataTypeStr=Inherit: Inherit via back propagation
  Gain1 : Gain  Gain=5/9  SaturateOnIntegerOverflow=on  OutDataTypeStr=Inherit: Same as input  ParamDataTypeStr=Inherit: Same as input
  Sum : Sum  Inputs=+-  SaturateOnIntegerOverflow=on  InputSameDT=on  OutDataTypeStr=Inherit: Same as first input
  C : Outport
  wires:
  Constant/1 -> Sum/2
  Gain1/1 -> C/1
  Sum/1 -> Gain1/1
  F/1 -> Sum/1

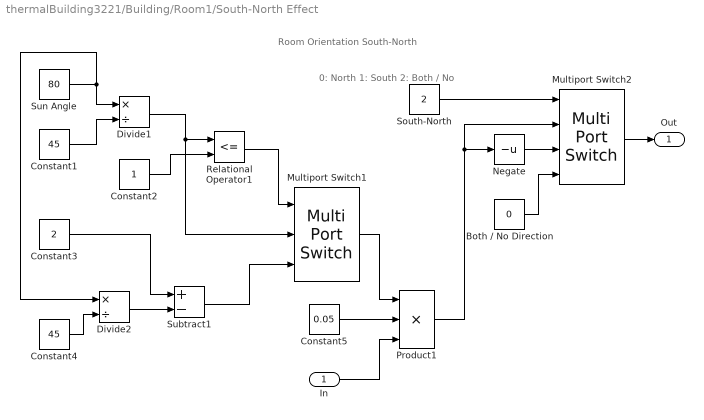
== system thermalBuilding3221/Building/Room1/South-North Effect ==
  note: 0: North
      | 1: South
      | 2: Both / No
  note: Room Orientation South-North
  In : Inport
  Both / No Direction : Constant  Value=0
  Constant1 : Constant  Value=45
  Constant2 : Constant
  Constant3 : Constant  Value=2
  Constant4 : Constant  Value=45
  Constant5 : Constant  Value=0.05
  Divide1 : Product  Inputs=*/
  Divide2 : Product  Inputs=*/
  Multiport Switch1 : MultiPortSwitch  DataPortOrder=Specify indices  Inputs=2  DataPortIndices={1,0}  DiagnosticForDefault=None
  Multiport Switch2 : MultiPortSwitch  DataPortOrder=Specify indices  Inputs=2  DataPortIndices={1,0,2}  DiagnosticForDefault=None
  Negate : UnaryMinus
  Product1 : Product  Inputs=3
  Relational Operator1 : RelationalOperator  Operator=<=  OutDataTypeStr=boolean
  South-North : Constant  Value=2
  Subtract1 : Sum  Inputs=+-
  Sun Angle : Constant  Value=80
  Out : Outport
  wires:
  Sun Angle/1 -> Divide2/1, Divide1/1
  Constant1/1 -> Divide1/2
  Divide1/1 -> Relational Operator1/1, Multiport Switch1/2
  Constant2/1 -> Relational Operator1/2
  Constant3/1 -> Subtract1/1
  Constant4/1 -> Divide2/2
  Divide2/1 -> Subtract1/2
  Relational Operator1/1 -> Multiport Switch1/1
  Subtract1/1 -> Multiport Switch1/3
  Multiport Switch1/1 -> Product1/1
  Constant5/1 -> Product1/2
  Product1/1 -> Multiport Switch2/2, Negate/1
  In/1 -> Product1/3
  South-North/1 -> Multiport Switch2/1
  Multiport Switch2/1 -> Out/1
  Negate/1 -> Multiport Switch2/3
  Both / No Direction/1 -> Multiport Switch2/4

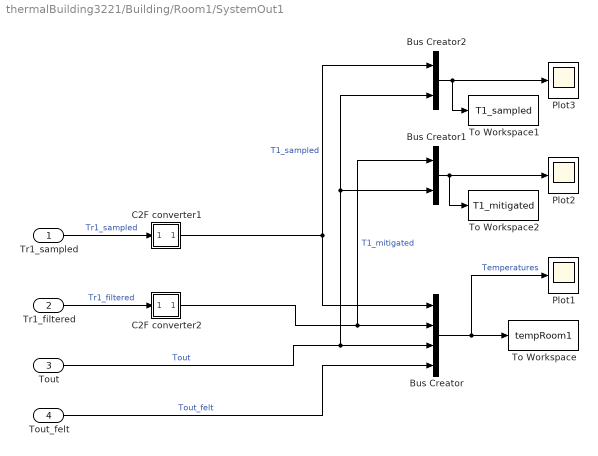
== system thermalBuilding3221/Building/Room1/SystemOut1 ==
  Tr1_sampled : Inport
  Tr1_filtered : Inport  Port=2
  Tout : Inport  Port=3
  Tout_felt : Inport  Port=4
  Bus Creator : BusCreator
  Bus Creator1 : BusCreator  Inputs=2
  Bus Creator2 : BusCreator  Inputs=2
  C2F converter1 : Subsystem  mask(F2C){}
      mask help:
      | Conversion from degrees Fahrenheit to degrees Celsius.
      |
      | F = C * (9/5) + 32;
      mask Display: image(imread('fahrenheit.jpg'))
  C2F converter2 : Subsystem  mask(F2C){}
      mask help:
      | Conversion from degrees Fahrenheit to degrees Celsius.
      |
      | F = C * (9/5) + 32;
      mask Display: image(imread('fahrenheit.jpg'))
  Plot1 : Scope
      settings: TickLabels=on  ShowLegends=on  TimeRange=50  YMin=0  YMax=40  SaveName=a1
  Plot2 : Scope
      settings: TickLabels=on  ShowLegends=on  TimeRange=50  YMin=0  YMax=40  SaveName=a4
  Plot3 : Scope
      settings: TickLabels=on  ShowLegends=on  TimeRange=50  YMin=0  YMax=40  SaveName=a5
  To Workspace : ToWorkspace  VariableName=tempRoom1  SampleTime=-1
  To Workspace1 : ToWorkspace  VariableName=T1_sampled  SampleTime=-1
  To Workspace2 : ToWorkspace  VariableName=T1_mitigated  SampleTime=-1
  wires:
  Bus Creator/1 -> Plot1/1, To Workspace/1  "Temperatures"
  Tr1_sampled/1 -> C2F converter1/1(F)  "Tr1_sampled"
  Tout/1 -> Bus Creator/3, Bus Creator2/2, Bus Creator1/2  "Tout"
  Tout_felt/1 -> Bus Creator/4  "Tout_felt"
  Tr1_filtered/1 -> C2F converter2/1(F)  "Tr1_filtered"
  Bus Creator2/1 -> To Workspace1/1, Plot3/1
  Bus Creator1/1 -> To Workspace2/1, Plot2/1
  C2F converter1/1(C) -> Bus Creator2/1, Bus Creator/1  "T1_sampled"
  C2F converter2/1(C) -> Bus Creator/2, Bus Creator1/1  "T1_mitigated"

== system thermalBuilding3221/Building/Room1/Temperature Sensor1 ==
  note: Temperature Sensor Subsystem
  In : Inport
  Add : Sum  Inputs=++|
  Constant : Constant  Value=0
  Out : Outport
  wires:
  In/1 -> Add/2
  Add/1 -> Out/1
  Constant/1 -> Add/1

== system thermalBuilding3221/Building/Room2/C2F converter1 ==
  F : Inport
  Constant1 : Constant  Value=32  OutDataTypeStr=Inherit: Inherit via back propagation
  Gain : Gain  Gain=9/5  SaturateOnIntegerOverflow=on  OutDataTypeStr=Inherit: Same as input  ParamDataTypeStr=Inherit: Same as input
  Sum1 : Sum  SaturateOnIntegerOverflow=on  InputSameDT=on  OutDataTypeStr=Inherit: Same as first input
  C : Outport
  wires:
  F/1 -> Gain/1
  Gain/1 -> Sum1/1
  Sum1/1 -> C/1
  Constant1/1 -> Sum1/2

== system thermalBuilding3221/Building/Room2/Controller2 ==
  note: Controller Subsystem
  note: Tset - Troom
  Sensor1 : Inport
  Data Store Write1 : DataStoreWrite  DataStoreName=RoC2
  Data Store Write2 : DataStoreWrite  DataStoreName=Tr2
  Filter : Subsystem
  Negate : UnaryMinus
  Reference Temperature : Subsystem
  Relay1 : Relay  OnSwitchValue=5*(5/9)  OffSwitchValue=0
  Relay2 : Relay  OnSwitchValue=5*(5/9)  OffSwitchValue=0
  RoC2 : Subsystem
  Sum : Sum  Inputs=-+|  SaturateOnIntegerOverflow=on  InputSameDT=on  OutDataTypeStr=Inherit: Same as first input
  Heater2 : Outport
  Cooler2 : Outport  Port=2
  FilterOut : Outport  Port=3
  wires:
  Reference Temperature/1(Tset) -> Sum/2
  Relay1/1 -> Heater2/1
  Relay2/1 -> Cooler2/1
  Negate/1 -> Relay2/1
  Sum/1 -> Relay1/1, Negate/1  "Tdiff"
  RoC2/1(Out1) -> Data Store Write1/1
  Sensor1/1 -> Filter/1(In1), RoC2/1(In1)
  Filter/1(Out1) -> Sum/1, Data Store Write2/1, FilterOut/1

== system thermalBuilding3221/Building/Room2/East-West Effect ==
  note: 0: West
      | 1: East
      | 2: Both / No
  note: Room Orientation East-West
  In : Inport
  Both / No Direction : Constant  Value=0
  Constant1 : Constant  Value=0.05
  East-West : Constant  Value=2
  From Workspace1 : FromWorkspace  VariableName=east  SampleTime=0
  From Workspace2 : FromWorkspace  VariableName=west  SampleTime=0
  Multiport Switch1 : MultiPortSwitch  DataPortOrder=Specify indices  Inputs=2  DataPortIndices={1,0,2}  DiagnosticForDefault=None
  Product1 : Product  Inputs=3
  Scope : Scope  NumInputPorts=2
      settings: YMin=-5~-5  YMax=5~5
  Out : Outport
  wires:
  From Workspace1/1 -> Scope/1, Multiport Switch1/2
  East-West/1 -> Multiport Switch1/1
  Product1/1 -> Out/1
  From Workspace2/1 -> Scope/2, Multiport Switch1/3
  Both / No Direction/1 -> Multiport Switch1/4
  Constant1/1 -> Product1/2
  In/1 -> Product1/3
  Multiport Switch1/1 -> Product1/1

== system thermalBuilding3221/Building/Room2/F2C   converter1 ==
  F : Inport
  Constant : Constant  Value=32  OutDataTypeStr=Inherit: Inherit via back propagation
  Gain1 : Gain  Gain=5/9  SaturateOnIntegerOverflow=on  OutDataTypeStr=Inherit: Same as input  ParamDataTypeStr=Inherit: Same as input
  Sum : Sum  Inputs=+-  SaturateOnIntegerOverflow=on  InputSameDT=on  OutDataTypeStr=Inherit: Same as first input
  C : Outport
  wires:
  Constant/1 -> Sum/2
  Gain1/1 -> C/1
  Sum/1 -> Gain1/1
  F/1 -> Sum/1

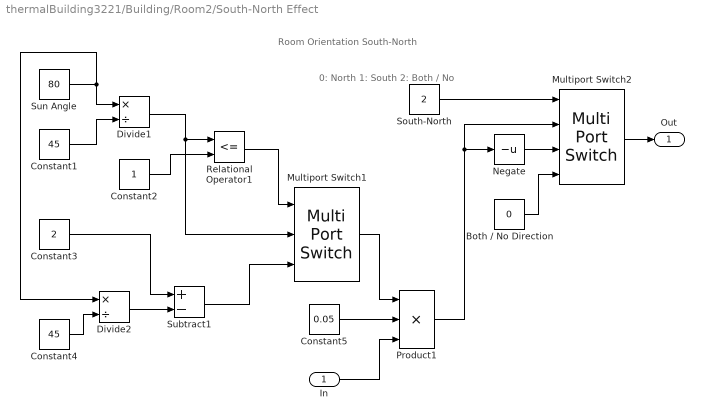
== system thermalBuilding3221/Building/Room2/South-North Effect ==
  note: 0: North
      | 1: South
      | 2: Both / No
  note: Room Orientation South-North
  In : Inport
  Both / No Direction : Constant  Value=0
  Constant1 : Constant  Value=45
  Constant2 : Constant
  Constant3 : Constant  Value=2
  Constant4 : Constant  Value=45
  Constant5 : Constant  Value=0.05
  Divide1 : Product  Inputs=*/
  Divide2 : Product  Inputs=*/
  Multiport Switch1 : MultiPortSwitch  DataPortOrder=Specify indices  Inputs=2  DataPortIndices={1,0}  DiagnosticForDefault=None
  Multiport Switch2 : MultiPortSwitch  DataPortOrder=Specify indices  Inputs=2  DataPortIndices={1,0,2}  DiagnosticForDefault=None
  Negate : UnaryMinus
  Product1 : Product  Inputs=3
  Relational Operator1 : RelationalOperator  Operator=<=  OutDataTypeStr=boolean
  South-North : Constant  Value=2
  Subtract1 : Sum  Inputs=+-
  Sun Angle : Constant  Value=80
  Out : Outport
  wires:
  Sun Angle/1 -> Divide2/1, Divide1/1
  Constant1/1 -> Divide1/2
  Divide1/1 -> Relational Operator1/1, Multiport Switch1/2
  Constant2/1 -> Relational Operator1/2
  Constant3/1 -> Subtract1/1
  Constant4/1 -> Divide2/2
  Divide2/1 -> Subtract1/2
  Relational Operator1/1 -> Multiport Switch1/1
  Subtract1/1 -> Multiport Switch1/3
  Multiport Switch1/1 -> Product1/1
  Constant5/1 -> Product1/2
  Product1/1 -> Multiport Switch2/2, Negate/1
  In/1 -> Product1/3
  South-North/1 -> Multiport Switch2/1
  Multiport Switch2/1 -> Out/1
  Negate/1 -> Multiport Switch2/3
  Both / No Direction/1 -> Multiport Switch2/4

== system thermalBuilding3221/Building/Room2/SystemOut2 ==
  T2_sampled : Inport
  T2_filtered : Inport  Port=2
  Tout : Inport  Port=3
  Tout_felt : Inport  Port=4
  Bus Creator : BusCreator
  Bus Creator1 : BusCreator  Inputs=2
  Bus Creator2 : BusCreator  Inputs=2
  C2F converter1 : Subsystem  mask(F2C){}
      mask help:
      | Conversion from degrees Fahrenheit to degrees Celsius.
      |
      | F = C * (9/5) + 32;
      mask Display: image(imread('fahrenheit.jpg'))
  C2F converter2 : Subsystem  mask(F2C){}
      mask help:
      | Conversion from degrees Fahrenheit to degrees Celsius.
      |
      | F = C * (9/5) + 32;
      mask Display: image(imread('fahrenheit.jpg'))
  Plot1 : Scope
      settings: TickLabels=on  ShowLegends=on  TimeRange=50  YMin=0  YMax=40  SaveName=a1
  Plot2 : Scope
      settings: TickLabels=on  ShowLegends=on  TimeRange=50  YMin=0  YMax=40  SaveName=a4
  Plot3 : Scope
      settings: TickLabels=on  ShowLegends=on  TimeRange=24  YMin=51  YMax=74  SaveName=a5
  To Workspace : ToWorkspace  VariableName=tempRoom2  SampleTime=-1
  To Workspace1 : ToWorkspace  VariableName=T2_sampled  SampleTime=-1
  To Workspace2 : ToWorkspace  VariableName=T2_mitigated  SampleTime=-1
  wires:
  Bus Creator/1 -> Plot1/1, To Workspace/1  "Temperatures"
  T2_sampled/1 -> C2F converter1/1(F)  "T1_sampled"
  Tout/1 -> Bus Creator/3, Bus Creator2/2, Bus Creator1/2  "Tout"
  Tout_felt/1 -> Bus Creator/4  "Tout_felt"
  T2_filtered/1 -> C2F converter2/1(F)  "T2_filtered"
  Bus Creator2/1 -> To Workspace1/1, Plot3/1
  Bus Creator1/1 -> To Workspace2/1, Plot2/1
  C2F converter1/1(C) -> Bus Creator2/1, Bus Creator/1  "T2_sampled"
  C2F converter2/1(C) -> Bus Creator/2, Bus Creator1/1  "T2_mitigated"

== system thermalBuilding3221/Building/Room2/Temperature Sensor2 ==
  note: Temperature Sensor Subsystem
  In : Inport
  Multiport Switch2 : MultiPortSwitch  DataPortOrder=Specify indices  Inputs=2  DataPortIndices={1,0}  DiagnosticForDefault=None
  Plot1 : Scope  NumInputPorts=2
      settings: TickLabels=on  ShowLegends=on  TimeRange=50  YMin=0~-5  YMax=40~5  SaveName=a
  Sample & Hold : Subsystem
  Sample and Hold : dspsigops/Sample and Hold  trig=Rising edge  initCond=0  latchinput=off
  Save time : Subsystem
  Single-Sample-Spike : Subsystem
  Spike and Stay width : Constant  Value=80/(100*stepSize)
  Sum : Sum  Inputs=-+|
  Timer : Subsystem
  Out : Outport
  wires:
  Save time/1(t) -> Sample & Hold/1(In1)
  Timer/1(time()) -> Save time/2(time()), Sample & Hold/2(In2)
  Sample & Hold/1(Out1) -> Multiport Switch2/1, Plot1/1, Sample and Hold/Trigger
  Spike and Stay width/1 -> Sample & Hold/3(In3)
  Single-Sample-Spike/1(Out) -> Sum/1, Save time/1(trigger)
  Multiport Switch2/1 -> Out/1, Plot1/2
  Sample and Hold/1 -> Multiport Switch2/2
  Sum/1 -> Multiport Switch2/3, Sample and Hold/1
  In/1 -> Sum/2

== system thermalBuilding3221/Building/Room3/C2F converter1 ==
  F : Inport
  Constant1 : Constant  Value=32  OutDataTypeStr=Inherit: Inherit via back propagation
  Gain : Gain  Gain=9/5  SaturateOnIntegerOverflow=on  OutDataTypeStr=Inherit: Same as input  ParamDataTypeStr=Inherit: Same as input
  Sum1 : Sum  SaturateOnIntegerOverflow=on  InputSameDT=on  OutDataTypeStr=Inherit: Same as first input
  C : Outport
  wires:
  F/1 -> Gain/1
  Gain/1 -> Sum1/1
  Sum1/1 -> C/1
  Constant1/1 -> Sum1/2

== system thermalBuilding3221/Building/Room3/C2F converter2 ==
  F : Inport
  Constant1 : Constant  Value=32  OutDataTypeStr=Inherit: Inherit via back propagation
  Gain : Gain  Gain=9/5  SaturateOnIntegerOverflow=on  OutDataTypeStr=Inherit: Same as input  ParamDataTypeStr=Inherit: Same as input
  Sum1 : Sum  SaturateOnIntegerOverflow=on  InputSameDT=on  OutDataTypeStr=Inherit: Same as first input
  C : Outport
  wires:
  F/1 -> Gain/1
  Gain/1 -> Sum1/1
  Sum1/1 -> C/1
  Constant1/1 -> Sum1/2

== system thermalBuilding3221/Building/Room3/Controller3 ==
  note: Controller Subsystem
  note: Tset - Troom
  Sensor3 : Inport
  Data Store Write1 : DataStoreWrite  DataStoreName=RoC3
  Data Store Write2 : DataStoreWrite  DataStoreName=Tr3
  Negate : UnaryMinus
  Reference Temperature : Subsystem
  Relay1 : Relay  OnSwitchValue=5*(5/9)  OffSwitchValue=0
  Relay2 : Relay  OnSwitchValue=5*(5/9)  OffSwitchValue=0
  RoC3 : Subsystem
  Sum : Sum  Inputs=-+|  SaturateOnIntegerOverflow=on  InputSameDT=on  OutDataTypeStr=Inherit: Same as first input
  Heater3 : Outport
  Cooler3 : Outport  Port=2
  FilterOut : Outport  Port=3
  wires:
  Reference Temperature/1(Tset) -> Sum/2
  Relay1/1 -> Heater3/1
  Relay2/1 -> Cooler3/1
  Negate/1 -> Relay2/1
  Sum/1 -> Relay1/1, Negate/1  "Tdiff"
  Sensor3/1 -> Sum/1, Data Store Write2/1, FilterOut/1, RoC3/1(In1)
  RoC3/1(Out1) -> Data Store Write1/1

== system thermalBuilding3221/Building/Room3/East-West Effect ==
  note: 0: West
      | 1: East
      | 2: Both / No
  note: Room Orientation East-West
  In : Inport
  Both / No Direction : Constant  Value=0
  Constant1 : Constant  Value=0.05
  East-West : Constant
  From Workspace1 : FromWorkspace  VariableName=east  SampleTime=0
  From Workspace2 : FromWorkspace  VariableName=west  SampleTime=0
  Multiport Switch1 : MultiPortSwitch  DataPortOrder=Specify indices  Inputs=2  DataPortIndices={1,0,2}  DiagnosticForDefault=None
  Product1 : Product  Inputs=3
  Scope : Scope  NumInputPorts=2
      settings: YMin=-5~-5  YMax=5~5
  Out : Outport
  wires:
  From Workspace1/1 -> Scope/1, Multiport Switch1/2
  East-West/1 -> Multiport Switch1/1
  Product1/1 -> Out/1
  From Workspace2/1 -> Scope/2, Multiport Switch1/3
  Both / No Direction/1 -> Multiport Switch1/4
  Constant1/1 -> Product1/2
  In/1 -> Product1/3
  Multiport Switch1/1 -> Product1/1

== system thermalBuilding3221/Building/Room3/F2C   converter1 ==
  F : Inport
  Constant : Constant  Value=32  OutDataTypeStr=Inherit: Inherit via back propagation
  Gain1 : Gain  Gain=5/9  SaturateOnIntegerOverflow=on  OutDataTypeStr=Inherit: Same as input  ParamDataTypeStr=Inherit: Same as input
  Sum : Sum  Inputs=+-  SaturateOnIntegerOverflow=on  InputSameDT=on  OutDataTypeStr=Inherit: Same as first input
  C : Outport
  wires:
  Constant/1 -> Sum/2
  Gain1/1 -> C/1
  Sum/1 -> Gain1/1
  F/1 -> Sum/1

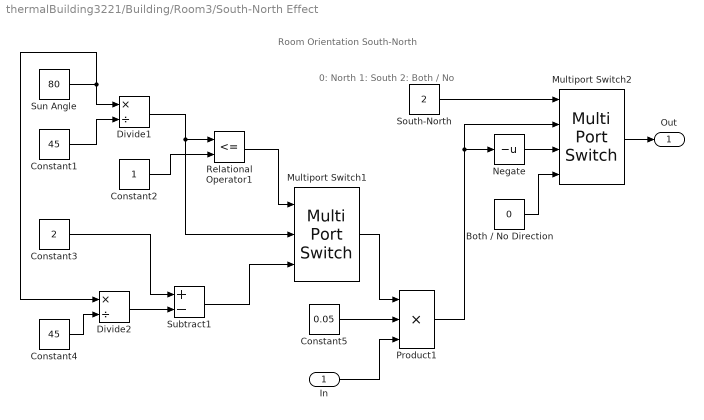
== system thermalBuilding3221/Building/Room3/South-North Effect ==
  note: 0: North
      | 1: South
      | 2: Both / No
  note: Room Orientation South-North
  In : Inport
  Both / No Direction : Constant  Value=0
  Constant1 : Constant  Value=45
  Constant2 : Constant
  Constant3 : Constant  Value=2
  Constant4 : Constant  Value=45
  Constant5 : Constant  Value=0.05
  Divide1 : Product  Inputs=*/
  Divide2 : Product  Inputs=*/
  Multiport Switch1 : MultiPortSwitch  DataPortOrder=Specify indices  Inputs=2  DataPortIndices={1,0}  DiagnosticForDefault=None
  Multiport Switch2 : MultiPortSwitch  DataPortOrder=Specify indices  Inputs=2  DataPortIndices={1,0,2}  DiagnosticForDefault=None
  Negate : UnaryMinus
  Product1 : Product  Inputs=3
  Relational Operator1 : RelationalOperator  Operator=<=  OutDataTypeStr=boolean
  South-North : Constant  Value=2
  Subtract1 : Sum  Inputs=+-
  Sun Angle : Constant  Value=80
  Out : Outport
  wires:
  Sun Angle/1 -> Divide2/1, Divide1/1
  Constant1/1 -> Divide1/2
  Divide1/1 -> Relational Operator1/1, Multiport Switch1/2
  Constant2/1 -> Relational Operator1/2
  Constant3/1 -> Subtract1/1
  Constant4/1 -> Divide2/2
  Divide2/1 -> Subtract1/2
  Relational Operator1/1 -> Multiport Switch1/1
  Subtract1/1 -> Multiport Switch1/3
  Multiport Switch1/1 -> Product1/1
  Constant5/1 -> Product1/2
  Product1/1 -> Multiport Switch2/2, Negate/1
  In/1 -> Product1/3
  South-North/1 -> Multiport Switch2/1
  Multiport Switch2/1 -> Out/1
  Negate/1 -> Multiport Switch2/3
  Both / No Direction/1 -> Multiport Switch2/4

== system thermalBuilding3221/Building/Room3/SystemOut3 ==
  Tr3_sampled : Inport
  Tr3_filtered : Inport  Port=2
  Tout : Inport  Port=3
  Tout_felt : Inport  Port=4
  Bus Creator : BusCreator
  Plot1 : Scope
      settings: TickLabels=on  ShowLegends=on  TimeRange=50  YMin=0  YMax=40  SaveName=a1
  To Workspace : ToWorkspace  VariableName=tempRoom3  SampleTime=-1
  wires:
  Bus Creator/1 -> Plot1/1, To Workspace/1  "Temperatures"
  Tr3_sampled/1 -> Bus Creator/1  "Tr3_sampled"
  Tout/1 -> Bus Creator/3  "Tout"
  Tout_felt/1 -> Bus Creator/4  "Tout_felt"
  Tr3_filtered/1 -> Bus Creator/2  "Tr3_filtered"

== system thermalBuilding3221/Building/Room3/Temperature Sensor3  ==
  note: Temperature Sensor Subsystem
  In : Inport
  Add : Sum  Inputs=++|
  Constant : Constant  Value=0
  Out : Outport
  wires:
  In/1 -> Add/2
  Add/1 -> Out/1
  Constant/1 -> Add/1

== system thermalBuilding3221/HVAC System/Cooler1/F2C   converter1 ==
  F : Inport
  Constant : Constant  Value=32  OutDataTypeStr=Inherit: Inherit via back propagation
  Gain1 : Gain  Gain=5/9  SaturateOnIntegerOverflow=on  OutDataTypeStr=Inherit: Same as input  ParamDataTypeStr=Inherit: Same as input
  Sum : Sum  Inputs=+-  SaturateOnIntegerOverflow=on  InputSameDT=on  OutDataTypeStr=Inherit: Same as first input
  C : Outport
  wires:
  Constant/1 -> Sum/2
  Gain1/1 -> C/1
  Sum/1 -> Gain1/1
  F/1 -> Sum/1

== system thermalBuilding3221/HVAC System/Cooler2/F2C   converter1 ==
  F : Inport
  Constant : Constant  Value=32  OutDataTypeStr=Inherit: Inherit via back propagation
  Gain1 : Gain  Gain=5/9  SaturateOnIntegerOverflow=on  OutDataTypeStr=Inherit: Same as input  ParamDataTypeStr=Inherit: Same as input
  Sum : Sum  Inputs=+-  SaturateOnIntegerOverflow=on  InputSameDT=on  OutDataTypeStr=Inherit: Same as first input
  C : Outport
  wires:
  Constant/1 -> Sum/2
  Gain1/1 -> C/1
  Sum/1 -> Gain1/1
  F/1 -> Sum/1
